simulink model "project"  (R2019a)
settings: Solver=FixedStepAuto  StartTime=0.0  StopTime=100  FixedStep=0.001  RelTol=1e-3
libraries: simulink x1
(part 1 of 2)
settings Model: Creator=shemmati  LastModifiedBy=shemmati
settings DataIOCC: ReturnWorkspaceOutputs=off
settings DebuggingCC: PregeneratedLibrarySubsystemCodeDiagnostic=none  ArithmeticOperatorsInVariantConditions=warning
settings SFSimCC: SimUseLocalCustomCode=off
settings RTWCC: RTWUseLocalCustomCode=off

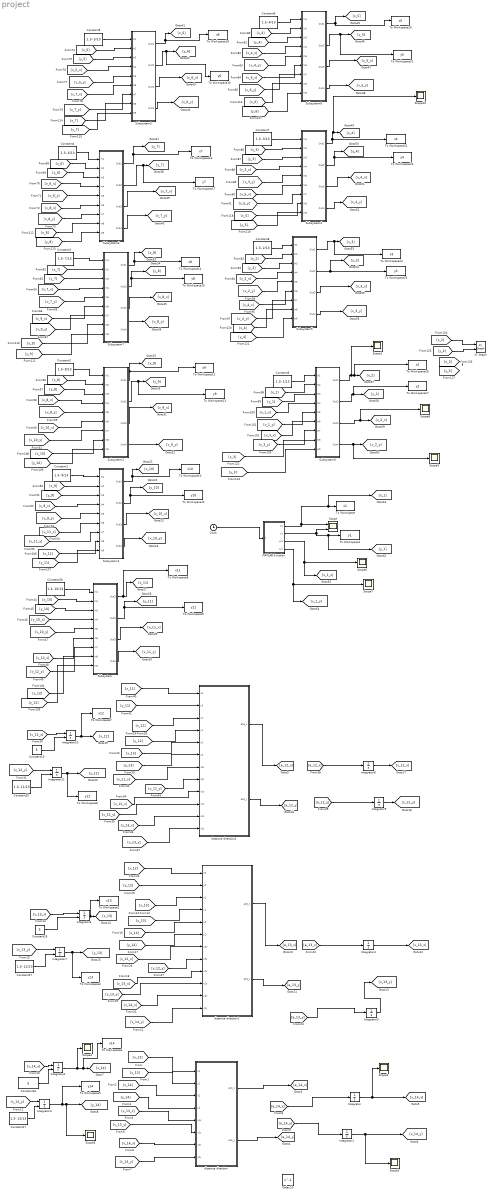
== system project ==
  Clock : Clock
  Constant1 : Constant  Value=1.3- 9/13
  Constant16 : Constant  Value=5
  Constant17 : Constant  Value=1.3- 13/13
  Constant18 : Constant  Value=5
  Constant19 : Constant  Value=5
  Constant2 : Constant  Value=1.3- 8/13
  Constant25 : Constant  Value=1.3- 11/13
  Constant27 : Constant  Value=1.3- 12/13
  Constant28 : Constant  Value=1.3- 10/13
  Constant3 : Constant  Value=1.3- 7/13
  Constant4 : Constant  Value=1.3- 6/13
  Constant5 : Constant  Value=1.3- 5/13
  Constant6 : Constant  Value=1.3- 4/13
  Constant7 : Constant  Value=1.3- 3/13
  Constant8 : Constant  Value=1.3- 2/13
  Constant9 : Constant  Value=1.3- 1/13
  Delay10 : Delay  DelayLength=1
  Integrator{,1,4..5,8..9} (6 alike) : Integrator
  Integrator{2..3,6..7,10..11} (6 alike) : Integrator  InitialConditionSource=external
  MATLAB Function : MATLAB Function  TreatAsAtomicUnit=on
  Scope : Scope  NumInputPorts=2
  Scope{1..10} (10 alike) : Scope
  Subsystem : Subsystem
  Subsystem1 : Subsystem
  Subsystem2 : Subsystem
  Subsystem3 : Subsystem
  Subsystem4 : Subsystem
  Subsystem5 : Subsystem
  Subsystem6 : Subsystem
  Subsystem7 : Subsystem
  Subsystem8 : Subsystem
  Subsystem9 : Subsystem
  To Workspace : ToWorkspace  VariableName=x1  SaveFormat=Timeseries  SampleTime=-1
  To Workspace1 : ToWorkspace  VariableName=y1  SaveFormat=Timeseries  SampleTime=-1
  To Workspace10 : ToWorkspace  VariableName=x10  SaveFormat=Timeseries  SampleTime=-1
  To Workspace11 : ToWorkspace  VariableName=y10  SaveFormat=Timeseries  SampleTime=-1
  To Workspace12 : ToWorkspace  VariableName=x9  SaveFormat=Timeseries  SampleTime=-1
  To Workspace13 : ToWorkspace  VariableName=y9  SaveFormat=Timeseries  SampleTime=-1
  To Workspace14 : ToWorkspace  VariableName=x8  SaveFormat=Timeseries  SampleTime=-1
  To Workspace15 : ToWorkspace  VariableName=y8  SaveFormat=Timeseries  SampleTime=-1
  To Workspace16 : ToWorkspace  VariableName=x7  SaveFormat=Timeseries  SampleTime=-1
  To Workspace17 : ToWorkspace  VariableName=y7  SaveFormat=Timeseries  SampleTime=-1
  To Workspace18 : ToWorkspace  VariableName=x6  SaveFormat=Timeseries  SampleTime=-1
  To Workspace19 : ToWorkspace  VariableName=y6  SaveFormat=Timeseries  SampleTime=-1
  To Workspace2 : ToWorkspace  VariableName=x13  SaveFormat=Timeseries  SampleTime=-1
  To Workspace20 : ToWorkspace  VariableName=x5  SaveFormat=Timeseries  SampleTime=-1
  To Workspace21 : ToWorkspace  VariableName=y5  SaveFormat=Timeseries  SampleTime=-1
  To Workspace22 : ToWorkspace  VariableName=x4  SaveFormat=Timeseries  SampleTime=-1
  To Workspace23 : ToWorkspace  VariableName=y4  SaveFormat=Timeseries  SampleTime=-1
  To Workspace24 : ToWorkspace  VariableName=x3  SaveFormat=Timeseries  SampleTime=-1
  To Workspace25 : ToWorkspace  VariableName=y3  SaveFormat=Timeseries  SampleTime=-1
  To Workspace26 : ToWorkspace  VariableName=x2  SaveFormat=Timeseries  SampleTime=-1
  To Workspace27 : ToWorkspace  VariableName=y2  SaveFormat=Timeseries  SampleTime=-1
  To Workspace3 : ToWorkspace  VariableName=y13  SaveFormat=Timeseries  SampleTime=-1
  To Workspace4 : ToWorkspace  VariableName=x14  SaveFormat=Timeseries  SampleTime=-1
  To Workspace5 : ToWorkspace  VariableName=y14  SaveFormat=Timeseries  SampleTime=-1
  To Workspace6 : ToWorkspace  VariableName=y12  SaveFormat=Timeseries  SampleTime=-1
  To Workspace7 : ToWorkspace  VariableName=x12  SaveFormat=Timeseries  SampleTime=-1
  To Workspace8 : ToWorkspace  VariableName=x11  SaveFormat=Timeseries  SampleTime=-1
  To Workspace9 : ToWorkspace  VariableName=y11  SaveFormat=Timeseries  SampleTime=-1
  XY Graph : simulink/Sinks/XY Graph  xmin=-20  xmax=20  ymin=-20  ymax=20  st=-1
  distance direction : MATLAB Function  TreatAsAtomicUnit=on
  distance direction1 : MATLAB Function  TreatAsAtomicUnit=on
  distance direction2 : MATLAB Function  TreatAsAtomicUnit=on
  wires:
  [x_13] -> distance direction/1(x1)
  [y_13] -> distance direction/2(y1)
  [x_14] -> distance direction/3(x2)
  [y_14] -> distance direction/4(y2)
  [v_14_x] -> Integrator2/1
  Constant16/1 -> Integrator2/2
  [v_14_y] -> Integrator3/1
  Constant17/1 -> Integrator3/2
  [x_13] -> distance direction1/3(x1)
  distance direction1/2(a13_y) -> [a_13_y]
  [v_14_x] -> distance direction1/11(v2x)
  [v_14_y] -> distance direction1/12(v2y)
  Integrator5/1 -> [v_13_y]
  Integrator4/1 -> [v_13_x]
  [v_13_y] -> distance direction1/10(v1y)
  [v_13_x] -> distance direction1/9(v1x)
  distance direction1/1(a13_x) -> [a_13_x]
  [y_14] -> distance direction1/6(y2)
  [y_13] -> distance direction1/4(y1)
  [v_13_y] -> Integrator7/1
  [v_13_x] -> Integrator6/1
  Constant18/1 -> Integrator6/2
  Constant27/1 -> Integrator7/2
  Integrator6/1 -> To Workspace2/1, [x_13]
  [x_14] -> distance direction1/5(x2)
  [x_12] -> distance direction1/1(x0)
  [y_12] -> distance direction1/2(y0)
  [v_12_x] -> distance direction1/7(v0x)
  [v_12_y] -> distance direction1/8(v0y)
  Integrator10/1 -> To Workspace7/1, [x_12]
  [x_13] -> distance direction2/5(x2)
  Integrator11/1 -> To Workspace6/1, [y_12]
  [v_12_x] -> Integrator10/1
  [y_13] -> distance direction2/6(y2)
  Constant25/1 -> Integrator11/2
  [v_12_y] -> Integrator11/1
  [x_11] -> distance direction2/1(x0)
  [v_11_x] -> distance direction2/7(v0x)
  Constant19/1 -> Integrator10/2
  [v_12_x] -> distance direction2/9(v1x)
  distance direction2/1(a13_x) -> [a_12_x]
  Integrator8/1 -> [v_12_x]
  Integrator9/1 -> [v_12_y]
  [v_12_y] -> distance direction2/10(v1y)
  distance direction2/2(a13_y) -> [a_12_y]
  [v_13_y] -> distance direction2/12(v2y)
  [y_11] -> distance direction2/2(y0)
  [x_12] -> distance direction2/3(x1)
  [v_11_y] -> distance direction2/8(v0y)
  [y_12] -> distance direction2/4(y1)
  [v_13_x] -> distance direction2/11(v2x)
  Constant28/1 -> Subsystem/1(In1)
  Subsystem/1(Out1) -> To Workspace8/1, [x_11]
  Subsystem/2(Out2) -> To Workspace9/1, [y_11]
  Subsystem/3(Out3) -> [v_11_x]
  Subsystem/4(Out4) -> [v_11_y]
  [x_10] -> Subsystem/2(In2)
  [y_10] -> Subsystem/3(In3)
  [v_10_x] -> Subsystem/4(In4)
  [v_10_y] -> Subsystem/5(In5)
  [v_12_x] -> Subsystem/6(In6)
  [v_12_y] -> Subsystem/7(In7)
  Subsystem1/4(Out4) -> [v_10_y]
  Subsystem1/1(Out1) -> To Workspace10/1, [x_10]
  Subsystem1/3(Out3) -> [v_10_x]
  Subsystem1/2(Out2) -> To Workspace11/1, [y_10]
  [v_11_y] -> Subsystem1/7(In7)
  Subsystem2/4(Out4) -> [v_9_y]
  Subsystem2/2(Out2) -> To Workspace13/1, [y_9]
  Subsystem2/3(Out3) -> [v_9_x]
  Subsystem2/1(Out1) -> To Workspace12/1, [x_9]
  Subsystem7/2(Out2) -> To Workspace15/1, [y_8]
  Subsystem7/4(Out4) -> [v_8_y]
  Subsystem7/3(Out3) -> [v_8_x]
  Subsystem7/1(Out1) -> To Workspace14/1, [x_8]
  Subsystem6/1(Out1) -> To Workspace16/1, [x_7]
  Subsystem6/2(Out2) -> To Workspace17/1, [y_7]
  Subsystem6/4(Out4) -> [v_7_y]
  Subsystem6/3(Out3) -> [v_7_x]
  Subsystem3/3(Out3) -> [v_6_x]
  Subsystem3/2(Out2) -> To Workspace19/1, [y_6]
  Subsystem3/1(Out1) -> To Workspace18/1, [x_6]
  Subsystem3/4(Out4) -> [v_6_y]
  Subsystem8/3(Out3) -> [v_5_x]
  Subsystem8/2(Out2) -> To Workspace21/1, [y_5]
  Subsystem8/1(Out1) -> [x_5], To Workspace20/1
  Subsystem8/4(Out4) -> [v_5_y]
  Subsystem5/1(Out1) -> To Workspace24/1, [x_3]
  Subsystem5/2(Out2) -> [y_3], To Workspace25/1
  Subsystem5/3(Out3) -> [v_3_x]
  Subsystem5/4(Out4) -> [v_3_y]
  MATLAB Function/2(y1) -> Scope/2, [y_1], To Workspace1/1
  Clock/1 -> MATLAB Function/1(t)
  MATLAB Function/1(x1) -> [x_1], To Workspace/1, Scope/1
  MATLAB Function/4(vy1) -> [v_1_y], Scope7/1
  MATLAB Function/3(vx1) -> Scope6/1, [v_1_x]
  [x_12] -> Subsystem/8(In8)
  [y_12] -> Subsystem/9(In9)
  Constant1/1 -> Subsystem1/1(In1)
  [x_9] -> Subsystem1/2(In2)
  [y_9] -> Subsystem1/3(In3)
  [v_9_x] -> Subsystem1/4(In4)
  [v_9_y] -> Subsystem1/5(In5)
  [v_11_x] -> Subsystem1/6(In6)
  [x_11] -> Subsystem1/8(In8)
  [y_11] -> Subsystem1/9(In9)
  Constant2/1 -> Subsystem2/1(In1)
  [x_8] -> Subsystem2/2(In2)
  [y_8] -> Subsystem2/3(In3)
  [v_8_x] -> Subsystem2/4(In4)
  [v_8_y] -> Subsystem2/5(In5)
  [v_10_x] -> Subsystem2/6(In6)
  [v_10_y] -> Subsystem2/7(In7)
  [x_10] -> Subsystem2/8(In8)
  [y_10] -> Subsystem2/9(In9)
  Constant3/1 -> Subsystem7/1(In1)
  [x_7] -> Subsystem7/2(In2)
  [y_7] -> Subsystem7/3(In3)
  [v_7_x] -> Subsystem7/4(In4)
  [v_7_y] -> Subsystem7/5(In5)
  [v_9_x] -> Subsystem7/6(In6)
  [v_9_y] -> Subsystem7/7(In7)
  [x_9] -> Subsystem7/8(In8)
  [y_9] -> Subsystem7/9(In9)
  [y_8] -> Subsystem6/9(In9)
  [x_8] -> Subsystem6/8(In8)
  [v_8_y] -> Subsystem6/7(In7)
  [v_8_x] -> Subsystem6/6(In6)
  [v_6_y] -> Subsystem6/5(In5)
  [v_6_x] -> Subsystem6/4(In4)
  [y_6] -> Subsystem6/3(In3)
  [x_6] -> Subsystem6/2(In2)
  Constant4/1 -> Subsystem6/1(In1)
  Constant5/1 -> Subsystem3/1(In1)
  [x_5] -> Subsystem3/2(In2)
  [y_5] -> Subsystem3/3(In3)
  [v_5_x] -> Subsystem3/4(In4)
  [v_5_y] -> Subsystem3/5(In5)
  [v_7_x] -> Subsystem3/6(In6)
  [v_7_y] -> Subsystem3/7(In7)
  [x_7] -> Subsystem3/8(In8)
  [y_7] -> Subsystem3/9(In9)
  Constant6/1 -> Subsystem8/1(In1)
  [x_4] -> Subsystem8/2(In2)
  [y_4] -> Subsystem8/3(In3)
  [v_4_x] -> Subsystem8/4(In4)
  [v_4_y] -> Subsystem8/5(In5)
  [v_6_x] -> Subsystem8/6(In6)
  [v_6_y] -> Subsystem8/7(In7)
  [x_6] -> Subsystem8/8(In8)
  [y_6] -> Subsystem8/9(In9)
  Constant7/1 -> Subsystem4/1(In1)
  [x_3] -> Subsystem4/2(In2)
  [y_3] -> Subsystem4/3(In3)
  [v_3_x] -> Subsystem4/4(In4)
  [v_3_y] -> Subsystem4/5(In5)
  [v_5_x] -> Subsystem4/6(In6)
  [v_5_y] -> Subsystem4/7(In7)
  [x_5] -> Subsystem4/8(In8)
  [y_5] -> Subsystem4/9(In9)
  Subsystem4/1(Out1) -> To Workspace22/1, Scope10/1, [x_4]
  Subsystem4/2(Out2) -> [y_4], To Workspace23/1
  Subsystem4/3(Out3) -> [v_4_x]
  Subsystem4/4(Out4) -> [v_4_y]
  Constant8/1 -> Subsystem5/1(In1)
  [x_2] -> Subsystem5/2(In2)
  [y_2] -> Subsystem5/3(In3)
  [v_2_x] -> Subsystem5/4(In4)
  [v_2_y] -> Subsystem5/5(In5)
  [v_4_x] -> Subsystem5/6(In6)
  [v_4_y] -> Subsystem5/7(In7)
  [x_4] -> Subsystem5/8(In8)
  [y_4] -> Subsystem5/9(In9)
  Constant9/1 -> Subsystem9/1(In1)
  [x_1] -> Subsystem9/2(In2)
  [y_1] -> Subsystem9/3(In3)
  [v_1_x] -> Subsystem9/4(In4)
  [v_1_y] -> Subsystem9/5(In5)
  [v_3_x] -> Subsystem9/6(In6)
  [v_3_y] -> Subsystem9/7(In7)
  Subsystem9/1(Out1) -> Scope1/1, To Workspace26/1, [x_2]
  Subsystem9/2(Out2) -> To Workspace27/1, [y_2]
  Subsystem9/3(Out3) -> Scope8/1, [v_2_x]
  Subsystem9/4(Out4) -> Scope9/1, [v_2_y]
  [x_3] -> Subsystem9/8(In8)
  [y_3] -> Subsystem9/9(In9)
  distance direction/1(a14_x) -> [a_14_x]
  distance direction/2(a14_y) -> [a_14_y]
  [v_14_y] -> distance direction/8(v2y)
  [v_14_x] -> distance direction/7(v2x)
  [v_13_y] -> distance direction/6(v1y)
  [v_13_x] -> distance direction/5(v1x)
  [a_13_x] -> Integrator4/1
  Integrator2/1 -> Scope4/1, To Workspace4/1, [x_14]
  Integrator3/1 -> To Workspace5/1, Scope5/1, [y_14]
  Integrator/1 -> Scope2/1, [v_14_x]
  Integrator1/1 -> Scope3/1, [v_14_y]
  [a_13_y] -> Integrator5/1
  [a_12_y] -> Integrator9/1
  [a_12_x] -> Integrator8/1
  [a_14_x] -> Integrator/1
  [a_14_y] -> Integrator1/1
  Integrator7/1 -> To Workspace3/1, [y_13]
  [x_2] -> XY Graph/1
  [y_2] -> XY Graph/2
  [x_3] -> ?

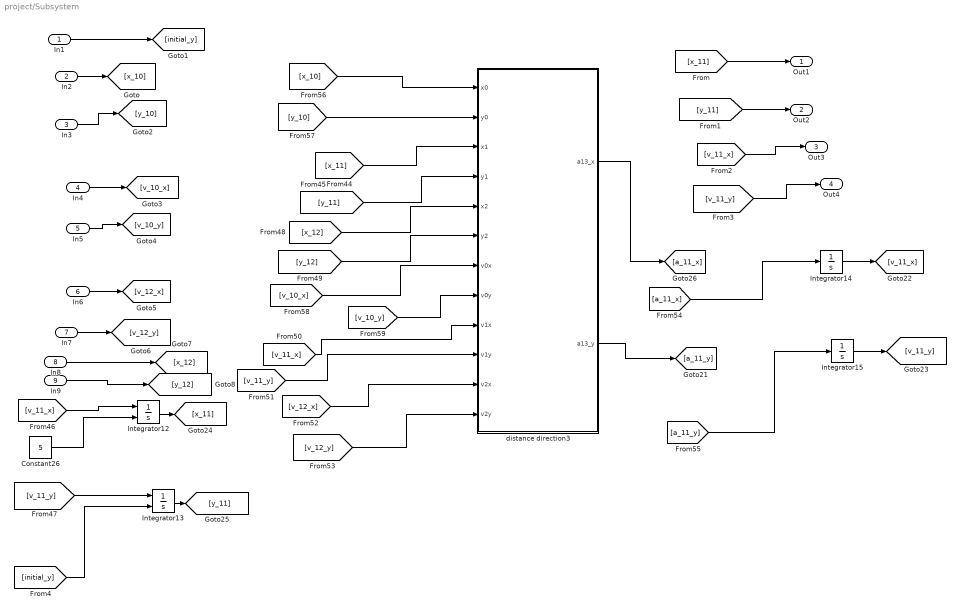
== system project/Subsystem ==
  In1 : Inport
  In2 : Inport  Port=2
  In3 : Inport  Port=3
  In4 : Inport  Port=4
  In5 : Inport  Port=5
  In6 : Inport  Port=6
  In7 : Inport  Port=7
  In8 : Inport  Port=8
  In9 : Inport  Port=9
  Constant26 : Constant  Value=5
  Integrator12 : Integrator  InitialConditionSource=external
  Integrator13 : Integrator  InitialConditionSource=external
  Integrator14 : Integrator
  Integrator15 : Integrator
  distance direction3 : MATLAB Function  TreatAsAtomicUnit=on
  Out1 : Outport
  Out2 : Outport  Port=2
  Out3 : Outport  Port=3
  Out4 : Outport  Port=4
  wires:
  distance direction3/1(a13_x) -> [a_11_x]
  Integrator15/1 -> [v_11_y]
  [v_12_y] -> distance direction3/12(v2y)
  [v_11_x] -> distance direction3/9(v1x)
  [v_10_x] -> distance direction3/7(v0x)
  distance direction3/2(a13_y) -> [a_11_y]
  [x_12] -> distance direction3/5(x2)
  [y_10] -> distance direction3/2(y0)
  [v_11_y] -> distance direction3/10(v1y)
  Constant26/1 -> Integrator12/2
  [v_12_x] -> distance direction3/11(v2x)
  [x_11] -> distance direction3/3(x1)
  [y_11] -> distance direction3/4(y1)
  Integrator12/1 -> [x_11]
  Integrator13/1 -> [y_11]
  [x_10] -> distance direction3/1(x0)
  [v_11_y] -> Integrator13/1
  Integrator14/1 -> [v_11_x]
  [initial_y] -> Integrator13/2
  [y_12] -> distance direction3/6(y2)
  [v_10_y] -> distance direction3/8(v0y)
  [v_11_x] -> Integrator12/1
  [x_11] -> Out1/1
  [y_11] -> Out2/1
  [v_11_x] -> Out3/1
  [v_11_y] -> Out4/1
  In1/1 -> [initial_y]
  In2/1 -> [x_10]
  In3/1 -> [y_10]
  In4/1 -> [v_10_x]
  In5/1 -> [v_10_y]
  In6/1 -> [v_12_x]
  In7/1 -> [v_12_y]
  In8/1 -> [x_12]
  In9/1 -> [y_12]
  [a_11_x] -> Integrator14/1
  [a_11_y] -> Integrator15/1

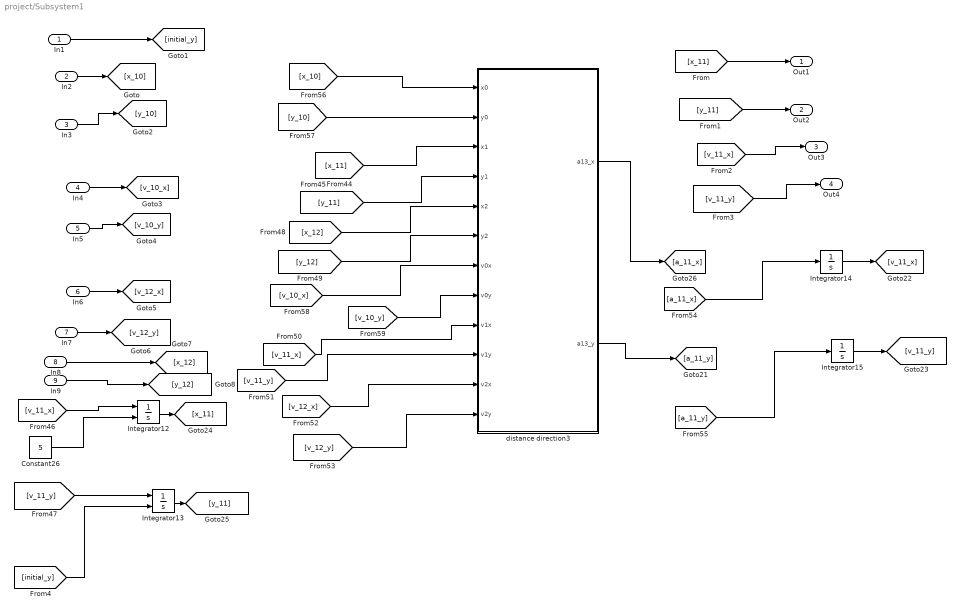
== system project/Subsystem1 ==
  In1 : Inport
  In2 : Inport  Port=2
  In3 : Inport  Port=3
  In4 : Inport  Port=4
  In5 : Inport  Port=5
  In6 : Inport  Port=6
  In7 : Inport  Port=7
  In8 : Inport  Port=8
  In9 : Inport  Port=9
  Constant26 : Constant  Value=5
  Integrator12 : Integrator  InitialConditionSource=external
  Integrator13 : Integrator  InitialConditionSource=external
  Integrator14 : Integrator
  Integrator15 : Integrator
  distance direction3 : MATLAB Function  TreatAsAtomicUnit=on
  Out1 : Outport
  Out2 : Outport  Port=2
  Out3 : Outport  Port=3
  Out4 : Outport  Port=4
  wires:
  distance direction3/1(a13_x) -> [a_11_x]
  Integrator15/1 -> [v_11_y]
  [v_12_y] -> distance direction3/12(v2y)
  [v_11_x] -> distance direction3/9(v1x)
  [v_10_x] -> distance direction3/7(v0x)
  distance direction3/2(a13_y) -> [a_11_y]
  [x_12] -> distance direction3/5(x2)
  [y_10] -> distance direction3/2(y0)
  [v_11_y] -> distance direction3/10(v1y)
  Constant26/1 -> Integrator12/2
  [v_12_x] -> distance direction3/11(v2x)
  [x_11] -> distance direction3/3(x1)
  [y_11] -> distance direction3/4(y1)
  Integrator12/1 -> [x_11]
  Integrator13/1 -> [y_11]
  [x_10] -> distance direction3/1(x0)
  [v_11_y] -> Integrator13/1
  Integrator14/1 -> [v_11_x]
  [initial_y] -> Integrator13/2
  [y_12] -> distance direction3/6(y2)
  [v_10_y] -> distance direction3/8(v0y)
  [v_11_x] -> Integrator12/1
  [x_11] -> Out1/1
  [y_11] -> Out2/1
  [v_11_x] -> Out3/1
  [v_11_y] -> Out4/1
  In1/1 -> [initial_y]
  In2/1 -> [x_10]
  In3/1 -> [y_10]
  In4/1 -> [v_10_x]
  In5/1 -> [v_10_y]
  In6/1 -> [v_12_x]
  In7/1 -> [v_12_y]
  In8/1 -> [x_12]
  In9/1 -> [y_12]
  [a_11_x] -> Integrator14/1
  [a_11_y] -> Integrator15/1

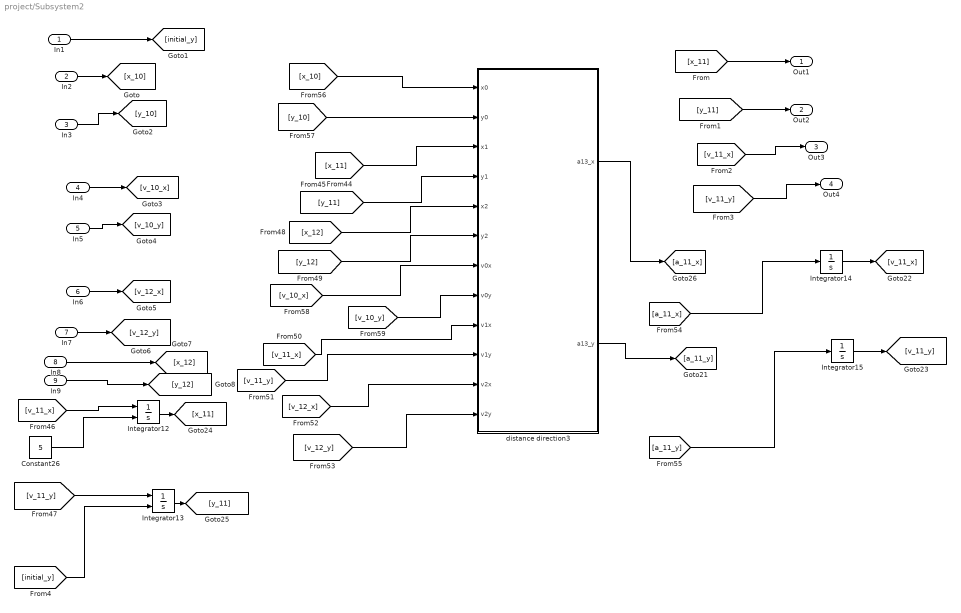
== system project/Subsystem2 ==
  In1 : Inport
  In2 : Inport  Port=2
  In3 : Inport  Port=3
  In4 : Inport  Port=4
  In5 : Inport  Port=5
  In6 : Inport  Port=6
  In7 : Inport  Port=7
  In8 : Inport  Port=8
  In9 : Inport  Port=9
  Constant26 : Constant  Value=5
  Integrator12 : Integrator  InitialConditionSource=external
  Integrator13 : Integrator  InitialConditionSource=external
  Integrator14 : Integrator
  Integrator15 : Integrator
  distance direction3 : MATLAB Function  TreatAsAtomicUnit=on
  Out1 : Outport
  Out2 : Outport  Port=2
  Out3 : Outport  Port=3
  Out4 : Outport  Port=4
  wires:
  distance direction3/1(a13_x) -> [a_11_x]
  Integrator15/1 -> [v_11_y]
  [v_12_y] -> distance direction3/12(v2y)
  [v_11_x] -> distance direction3/9(v1x)
  [v_10_x] -> distance direction3/7(v0x)
  distance direction3/2(a13_y) -> [a_11_y]
  [x_12] -> distance direction3/5(x2)
  [y_10] -> distance direction3/2(y0)
  [v_11_y] -> distance direction3/10(v1y)
  Constant26/1 -> Integrator12/2
  [v_12_x] -> distance direction3/11(v2x)
  [x_11] -> distance direction3/3(x1)
  [y_11] -> distance direction3/4(y1)
  Integrator12/1 -> [x_11]
  Integrator13/1 -> [y_11]
  [x_10] -> distance direction3/1(x0)
  [v_11_y] -> Integrator13/1
  Integrator14/1 -> [v_11_x]
  [initial_y] -> Integrator13/2
  [y_12] -> distance direction3/6(y2)
  [v_10_y] -> distance direction3/8(v0y)
  [v_11_x] -> Integrator12/1
  [x_11] -> Out1/1
  [y_11] -> Out2/1
  [v_11_x] -> Out3/1
  [v_11_y] -> Out4/1
  In1/1 -> [initial_y]
  In2/1 -> [x_10]
  In3/1 -> [y_10]
  In4/1 -> [v_10_x]
  In5/1 -> [v_10_y]
  In6/1 -> [v_12_x]
  In7/1 -> [v_12_y]
  In8/1 -> [x_12]
  In9/1 -> [y_12]
  [a_11_x] -> Integrator14/1
  [a_11_y] -> Integrator15/1

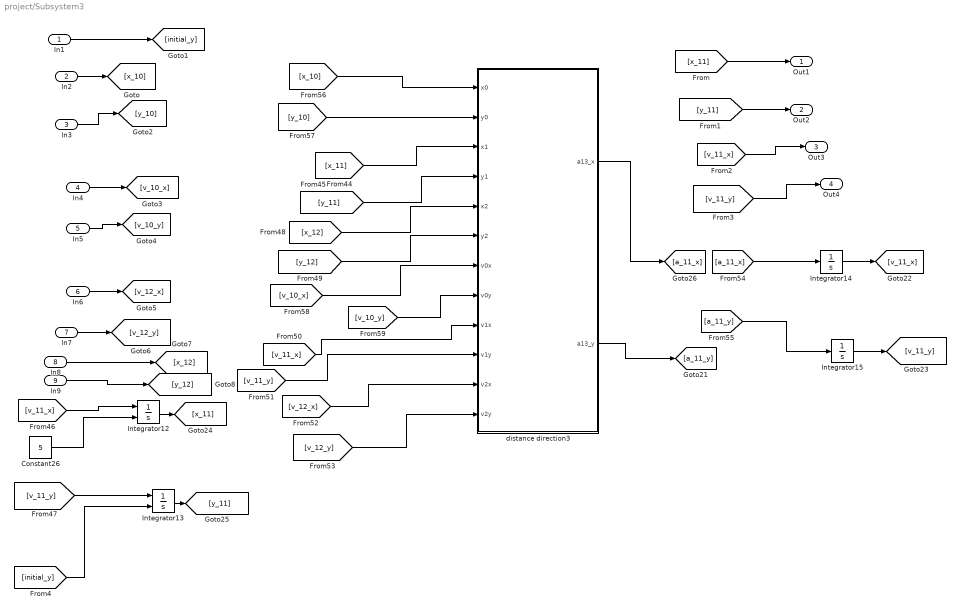
== system project/Subsystem3 ==
  In1 : Inport
  In2 : Inport  Port=2
  In3 : Inport  Port=3
  In4 : Inport  Port=4
  In5 : Inport  Port=5
  In6 : Inport  Port=6
  In7 : Inport  Port=7
  In8 : Inport  Port=8
  In9 : Inport  Port=9
  Constant26 : Constant  Value=5
  Integrator12 : Integrator  InitialConditionSource=external
  Integrator13 : Integrator  InitialConditionSource=external
  Integrator14 : Integrator
  Integrator15 : Integrator
  distance direction3 : MATLAB Function  TreatAsAtomicUnit=on
  Out1 : Outport
  Out2 : Outport  Port=2
  Out3 : Outport  Port=3
  Out4 : Outport  Port=4
  wires:
  distance direction3/1(a13_x) -> [a_11_x]
  Integrator15/1 -> [v_11_y]
  [v_12_y] -> distance direction3/12(v2y)
  [v_11_x] -> distance direction3/9(v1x)
  [v_10_x] -> distance direction3/7(v0x)
  distance direction3/2(a13_y) -> [a_11_y]
  [x_12] -> distance direction3/5(x2)
  [y_10] -> distance direction3/2(y0)
  [v_11_y] -> distance direction3/10(v1y)
  Constant26/1 -> Integrator12/2
  [v_12_x] -> distance direction3/11(v2x)
  [x_11] -> distance direction3/3(x1)
  [y_11] -> distance direction3/4(y1)
  Integrator12/1 -> [x_11]
  Integrator13/1 -> [y_11]
  [x_10] -> distance direction3/1(x0)
  [v_11_y] -> Integrator13/1
  Integrator14/1 -> [v_11_x]
  [initial_y] -> Integrator13/2
  [y_12] -> distance direction3/6(y2)
  [v_10_y] -> distance direction3/8(v0y)
  [v_11_x] -> Integrator12/1
  [x_11] -> Out1/1
  [y_11] -> Out2/1
  [v_11_x] -> Out3/1
  [v_11_y] -> Out4/1
  In1/1 -> [initial_y]
  In2/1 -> [x_10]
  In3/1 -> [y_10]
  In4/1 -> [v_10_x]
  In5/1 -> [v_10_y]
  In6/1 -> [v_12_x]
  In7/1 -> [v_12_y]
  In8/1 -> [x_12]
  In9/1 -> [y_12]
  [a_11_x] -> Integrator14/1
  [a_11_y] -> Integrator15/1

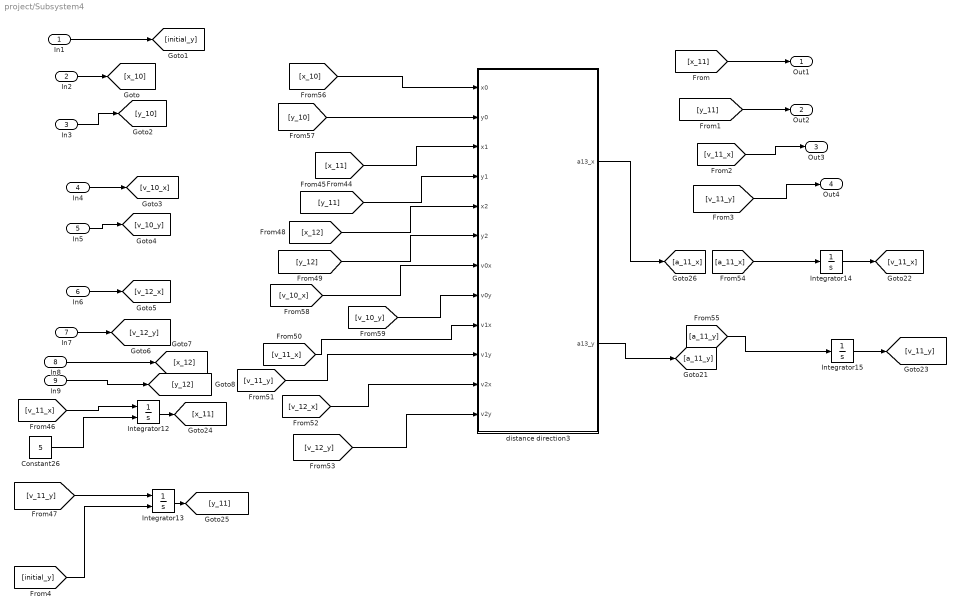
== system project/Subsystem4 ==
  In1 : Inport
  In2 : Inport  Port=2
  In3 : Inport  Port=3
  In4 : Inport  Port=4
  In5 : Inport  Port=5
  In6 : Inport  Port=6
  In7 : Inport  Port=7
  In8 : Inport  Port=8
  In9 : Inport  Port=9
  Constant26 : Constant  Value=5
  Integrator12 : Integrator  InitialConditionSource=external
  Integrator13 : Integrator  InitialConditionSource=external
  Integrator14 : Integrator
  Integrator15 : Integrator
  distance direction3 : MATLAB Function  TreatAsAtomicUnit=on
  Out1 : Outport
  Out2 : Outport  Port=2
  Out3 : Outport  Port=3
  Out4 : Outport  Port=4
  wires:
  distance direction3/1(a13_x) -> [a_11_x]
  Integrator15/1 -> [v_11_y]
  [v_12_y] -> distance direction3/12(v2y)
  [v_11_x] -> distance direction3/9(v1x)
  [v_10_x] -> distance direction3/7(v0x)
  distance direction3/2(a13_y) -> [a_11_y]
  [x_12] -> distance direction3/5(x2)
  [y_10] -> distance direction3/2(y0)
  [v_11_y] -> distance direction3/10(v1y)
  Constant26/1 -> Integrator12/2
  [v_12_x] -> distance direction3/11(v2x)
  [x_11] -> distance direction3/3(x1)
  [y_11] -> distance direction3/4(y1)
  Integrator12/1 -> [x_11]
  Integrator13/1 -> [y_11]
  [x_10] -> distance direction3/1(x0)
  [v_11_y] -> Integrator13/1
  Integrator14/1 -> [v_11_x]
  [initial_y] -> Integrator13/2
  [y_12] -> distance direction3/6(y2)
  [v_10_y] -> distance direction3/8(v0y)
  [v_11_x] -> Integrator12/1
  [x_11] -> Out1/1
  [y_11] -> Out2/1
  [v_11_x] -> Out3/1
  [v_11_y] -> Out4/1
  In1/1 -> [initial_y]
  In2/1 -> [x_10]
  In3/1 -> [y_10]
  In4/1 -> [v_10_x]
  In5/1 -> [v_10_y]
  In6/1 -> [v_12_x]
  In7/1 -> [v_12_y]
  In8/1 -> [x_12]
  In9/1 -> [y_12]
  [a_11_x] -> Integrator14/1
  [a_11_y] -> Integrator15/1

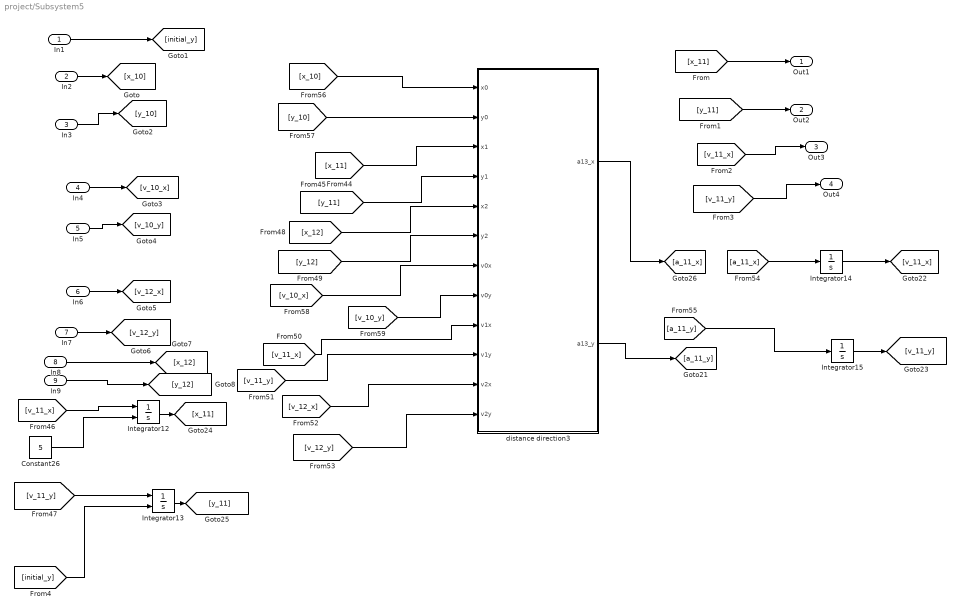
== system project/Subsystem5 ==
  In1 : Inport
  In2 : Inport  Port=2
  In3 : Inport  Port=3
  In4 : Inport  Port=4
  In5 : Inport  Port=5
  In6 : Inport  Port=6
  In7 : Inport  Port=7
  In8 : Inport  Port=8
  In9 : Inport  Port=9
  Constant26 : Constant  Value=5
  Integrator12 : Integrator  InitialConditionSource=external
  Integrator13 : Integrator  InitialConditionSource=external
  Integrator14 : Integrator
  Integrator15 : Integrator
  distance direction3 : MATLAB Function  TreatAsAtomicUnit=on
  Out1 : Outport
  Out2 : Outport  Port=2
  Out3 : Outport  Port=3
  Out4 : Outport  Port=4
  wires:
  distance direction3/1(a13_x) -> [a_11_x]
  Integrator15/1 -> [v_11_y]
  [v_12_y] -> distance direction3/12(v2y)
  [v_11_x] -> distance direction3/9(v1x)
  [v_10_x] -> distance direction3/7(v0x)
  distance direction3/2(a13_y) -> [a_11_y]
  [x_12] -> distance direction3/5(x2)
  [y_10] -> distance direction3/2(y0)
  [v_11_y] -> distance direction3/10(v1y)
  Constant26/1 -> Integrator12/2
  [v_12_x] -> distance direction3/11(v2x)
  [x_11] -> distance direction3/3(x1)
  [y_11] -> distance direction3/4(y1)
  Integrator12/1 -> [x_11]
  Integrator13/1 -> [y_11]
  [x_10] -> distance direction3/1(x0)
  [v_11_y] -> Integrator13/1
  Integrator14/1 -> [v_11_x]
  [initial_y] -> Integrator13/2
  [y_12] -> distance direction3/6(y2)
  [v_10_y] -> distance direction3/8(v0y)
  [v_11_x] -> Integrator12/1
  [x_11] -> Out1/1
  [y_11] -> Out2/1
  [v_11_x] -> Out3/1
  [v_11_y] -> Out4/1
  In1/1 -> [initial_y]
  In2/1 -> [x_10]
  In3/1 -> [y_10]
  In4/1 -> [v_10_x]
  In5/1 -> [v_10_y]
  In6/1 -> [v_12_x]
  In7/1 -> [v_12_y]
  In8/1 -> [x_12]
  In9/1 -> [y_12]
  [a_11_x] -> Integrator14/1
  [a_11_y] -> Integrator15/1

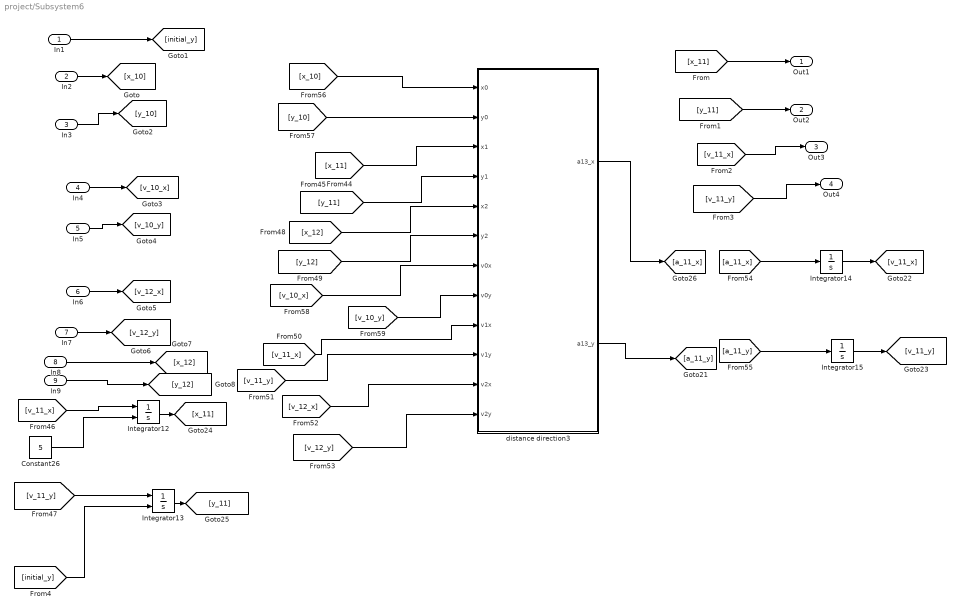
== system project/Subsystem6 ==
  In1 : Inport
  In2 : Inport  Port=2
  In3 : Inport  Port=3
  In4 : Inport  Port=4
  In5 : Inport  Port=5
  In6 : Inport  Port=6
  In7 : Inport  Port=7
  In8 : Inport  Port=8
  In9 : Inport  Port=9
  Constant26 : Constant  Value=5
  Integrator12 : Integrator  InitialConditionSource=external
  Integrator13 : Integrator  InitialConditionSource=external
  Integrator14 : Integrator
  Integrator15 : Integrator
  distance direction3 : MATLAB Function  TreatAsAtomicUnit=on
  Out1 : Outport
  Out2 : Outport  Port=2
  Out3 : Outport  Port=3
  Out4 : Outport  Port=4
  wires:
  distance direction3/1(a13_x) -> [a_11_x]
  Integrator15/1 -> [v_11_y]
  [v_12_y] -> distance direction3/12(v2y)
  [v_11_x] -> distance direction3/9(v1x)
  [v_10_x] -> distance direction3/7(v0x)
  distance direction3/2(a13_y) -> [a_11_y]
  [x_12] -> distance direction3/5(x2)
  [y_10] -> distance direction3/2(y0)
  [v_11_y] -> distance direction3/10(v1y)
  Constant26/1 -> Integrator12/2
  [v_12_x] -> distance direction3/11(v2x)
  [x_11] -> distance direction3/3(x1)
  [y_11] -> distance direction3/4(y1)
  Integrator12/1 -> [x_11]
  Integrator13/1 -> [y_11]
  [x_10] -> distance direction3/1(x0)
  [v_11_y] -> Integrator13/1
  Integrator14/1 -> [v_11_x]
  [initial_y] -> Integrator13/2
  [y_12] -> distance direction3/6(y2)
  [v_10_y] -> distance direction3/8(v0y)
  [v_11_x] -> Integrator12/1
  [x_11] -> Out1/1
  [y_11] -> Out2/1
  [v_11_x] -> Out3/1
  [v_11_y] -> Out4/1
  In1/1 -> [initial_y]
  In2/1 -> [x_10]
  In3/1 -> [y_10]
  In4/1 -> [v_10_x]
  In5/1 -> [v_10_y]
  In6/1 -> [v_12_x]
  In7/1 -> [v_12_y]
  In8/1 -> [x_12]
  In9/1 -> [y_12]
  [a_11_x] -> Integrator14/1
  [a_11_y] -> Integrator15/1

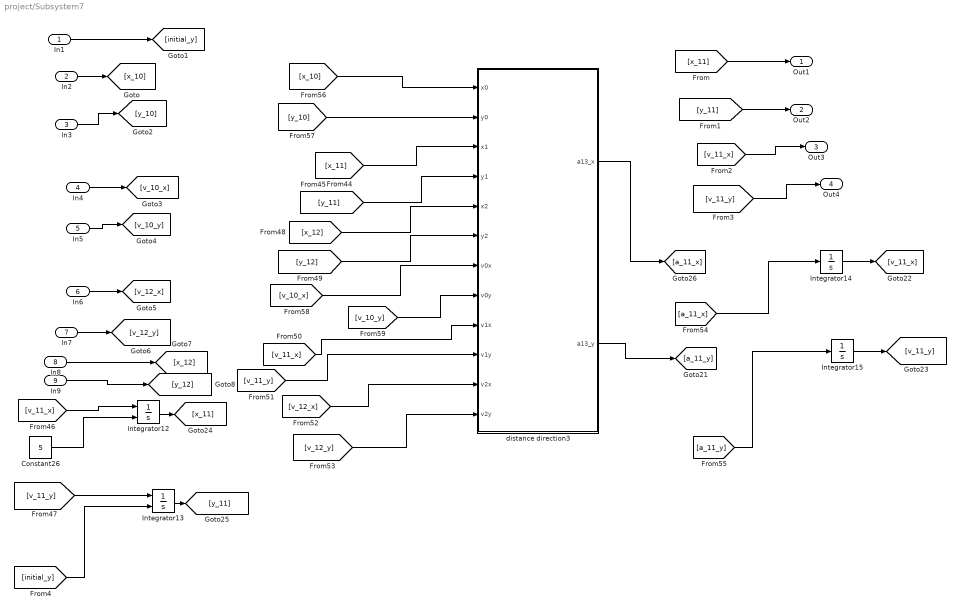
== system project/Subsystem7 ==
  In1 : Inport
  In2 : Inport  Port=2
  In3 : Inport  Port=3
  In4 : Inport  Port=4
  In5 : Inport  Port=5
  In6 : Inport  Port=6
  In7 : Inport  Port=7
  In8 : Inport  Port=8
  In9 : Inport  Port=9
  Constant26 : Constant  Value=5
  Integrator12 : Integrator  InitialConditionSource=external
  Integrator13 : Integrator  InitialConditionSource=external
  Integrator14 : Integrator
  Integrator15 : Integrator
  distance direction3 : MATLAB Function  TreatAsAtomicUnit=on
  Out1 : Outport
  Out2 : Outport  Port=2
  Out3 : Outport  Port=3
  Out4 : Outport  Port=4
  wires:
  distance direction3/1(a13_x) -> [a_11_x]
  Integrator15/1 -> [v_11_y]
  [v_12_y] -> distance direction3/12(v2y)
  [v_11_x] -> distance direction3/9(v1x)
  [v_10_x] -> distance direction3/7(v0x)
  distance direction3/2(a13_y) -> [a_11_y]
  [x_12] -> distance direction3/5(x2)
  [y_10] -> distance direction3/2(y0)
  [v_11_y] -> distance direction3/10(v1y)
  Constant26/1 -> Integrator12/2
  [v_12_x] -> distance direction3/11(v2x)
  [x_11] -> distance direction3/3(x1)
  [y_11] -> distance direction3/4(y1)
  Integrator12/1 -> [x_11]
  Integrator13/1 -> [y_11]
  [x_10] -> distance direction3/1(x0)
  [v_11_y] -> Integrator13/1
  Integrator14/1 -> [v_11_x]
  [initial_y] -> Integrator13/2
  [y_12] -> distance direction3/6(y2)
  [v_10_y] -> distance direction3/8(v0y)
  [v_11_x] -> Integrator12/1
  [x_11] -> Out1/1
  [y_11] -> Out2/1
  [v_11_x] -> Out3/1
  [v_11_y] -> Out4/1
  In1/1 -> [initial_y]
  In2/1 -> [x_10]
  In3/1 -> [y_10]
  In4/1 -> [v_10_x]
  In5/1 -> [v_10_y]
  In6/1 -> [v_12_x]
  In7/1 -> [v_12_y]
  In8/1 -> [x_12]
  In9/1 -> [y_12]
  [a_11_y] -> Integrator15/1
  [a_11_x] -> Integrator14/1

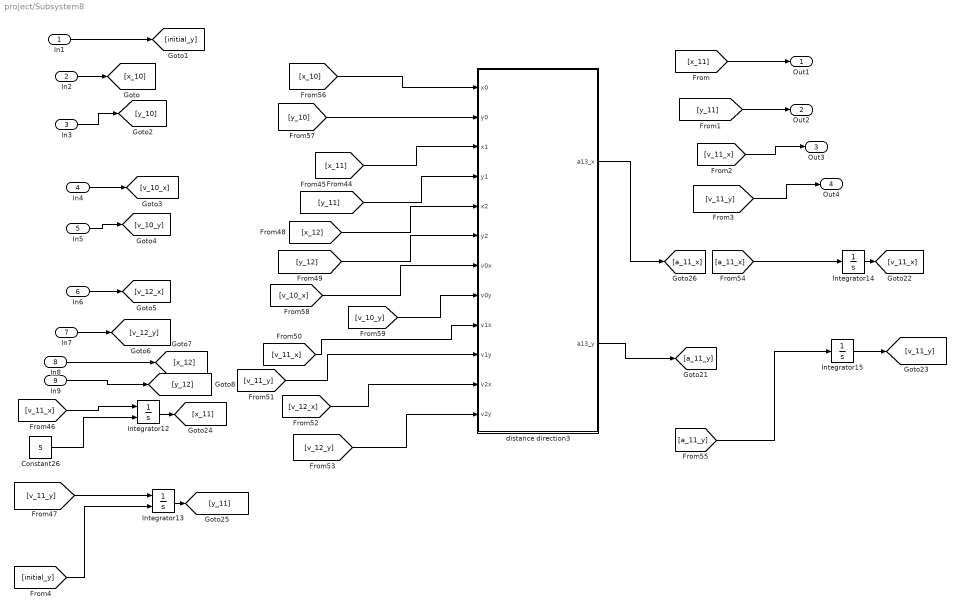
== system project/Subsystem8 ==
  In1 : Inport
  In2 : Inport  Port=2
  In3 : Inport  Port=3
  In4 : Inport  Port=4
  In5 : Inport  Port=5
  In6 : Inport  Port=6
  In7 : Inport  Port=7
  In8 : Inport  Port=8
  In9 : Inport  Port=9
  Constant26 : Constant  Value=5
  Integrator12 : Integrator  InitialConditionSource=external
  Integrator13 : Integrator  InitialConditionSource=external
  Integrator14 : Integrator
  Integrator15 : Integrator
  distance direction3 : MATLAB Function  TreatAsAtomicUnit=on
  Out1 : Outport
  Out2 : Outport  Port=2
  Out3 : Outport  Port=3
  Out4 : Outport  Port=4
  wires:
  distance direction3/1(a13_x) -> [a_11_x]
  Integrator15/1 -> [v_11_y]
  [v_12_y] -> distance direction3/12(v2y)
  [v_11_x] -> distance direction3/9(v1x)
  [v_10_x] -> distance direction3/7(v0x)
  distance direction3/2(a13_y) -> [a_11_y]
  [x_12] -> distance direction3/5(x2)
  [y_10] -> distance direction3/2(y0)
  [v_11_y] -> distance direction3/10(v1y)
  Constant26/1 -> Integrator12/2
  [v_12_x] -> distance direction3/11(v2x)
  [x_11] -> distance direction3/3(x1)
  [y_11] -> distance direction3/4(y1)
  Integrator12/1 -> [x_11]
  Integrator13/1 -> [y_11]
  [x_10] -> distance direction3/1(x0)
  [v_11_y] -> Integrator13/1
  Integrator14/1 -> [v_11_x]
  [initial_y] -> Integrator13/2
  [y_12] -> distance direction3/6(y2)
  [v_10_y] -> distance direction3/8(v0y)
  [v_11_x] -> Integrator12/1
  [x_11] -> Out1/1
  [y_11] -> Out2/1
  [v_11_x] -> Out3/1
  [v_11_y] -> Out4/1
  In1/1 -> [initial_y]
  In2/1 -> [x_10]
  In3/1 -> [y_10]
  In4/1 -> [v_10_x]
  In5/1 -> [v_10_y]
  In6/1 -> [v_12_x]
  In7/1 -> [v_12_y]
  In8/1 -> [x_12]
  In9/1 -> [y_12]
  [a_11_x] -> Integrator14/1
  [a_11_y] -> Integrator15/1

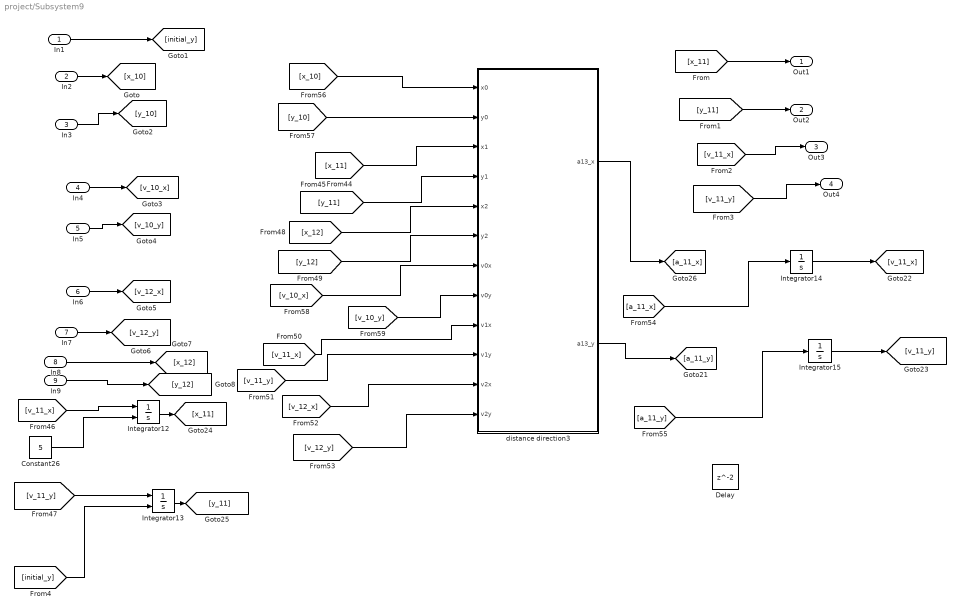
== system project/Subsystem9 ==
  In1 : Inport
  In2 : Inport  Port=2
  In3 : Inport  Port=3
  In4 : Inport  Port=4
  In5 : Inport  Port=5
  In6 : Inport  Port=6
  In7 : Inport  Port=7
  In8 : Inport  Port=8
  In9 : Inport  Port=9
  Constant26 : Constant  Value=5
  Delay : Delay
  Integrator12 : Integrator  InitialConditionSource=external
  Integrator13 : Integrator  InitialConditionSource=external
  Integrator14 : Integrator
  Integrator15 : Integrator
  distance direction3 : MATLAB Function  TreatAsAtomicUnit=on
  Out1 : Outport
  Out2 : Outport  Port=2
  Out3 : Outport  Port=3
  Out4 : Outport  Port=4
  wires:
  distance direction3/1(a13_x) -> [a_11_x]
  [v_12_y] -> distance direction3/12(v2y)
  [v_11_x] -> distance direction3/9(v1x)
  [v_10_x] -> distance direction3/7(v0x)
  distance direction3/2(a13_y) -> [a_11_y]
  [x_12] -> distance direction3/5(x2)
  [y_10] -> distance direction3/2(y0)
  [v_11_y] -> distance direction3/10(v1y)
  Constant26/1 -> Integrator12/2
  [v_12_x] -> distance direction3/11(v2x)
  [x_11] -> distance direction3/3(x1)
  [y_11] -> distance direction3/4(y1)
  Integrator12/1 -> [x_11]
  Integrator13/1 -> [y_11]
  [x_10] -> distance direction3/1(x0)
  [v_11_y] -> Integrator13/1
  [initial_y] -> Integrator13/2
  [y_12] -> distance direction3/6(y2)
  [v_10_y] -> distance direction3/8(v0y)
  [v_11_x] -> Integrator12/1
  [x_11] -> Out1/1
  [y_11] -> Out2/1
  [v_11_x] -> Out3/1
  [v_11_y] -> Out4/1
  In1/1 -> [initial_y]
  In2/1 -> [x_10]
  In3/1 -> [y_10]
  In4/1 -> [v_10_x]
  In5/1 -> [v_10_y]
  In6/1 -> [v_12_x]
  In7/1 -> [v_12_y]
  In8/1 -> [x_12]
  In9/1 -> [y_12]
  Integrator14/1 -> [v_11_x]
  Integrator15/1 -> [v_11_y]
  [a_11_x] -> Integrator14/1
  [a_11_y] -> Integrator15/1

== matlab function project/distance direction ==
  data: x1 input; y1 input; x2 input; y2 input; v1x input; v1y input; a14_x output size=1; a14_y output size=1; v2x input; v2y input
function [a14_x, a14_y] = fcn(x1, y1, x2, y2, v1x,v1y, v2x, v2y)




m=1/10;

k_s= 10;

k_d= 1;

L_r= 1/13;


distance= sqrt((x1-x2)^2 + (y1-y2)^2);


theta_after= atan2((y2-y1),(x2-x1));
% if x1~=x2
% theta_after= atan((y1-y2)/(x1-x2))
% else
% theta_after= 3.14/2;
% end


f_spring_x_13_14= -k_s* (distance - L_r)* cos(theta_after);

f_spring_y_13_14= -k_s* (distance - L_r)* sin(theta_after);



theta_damper_after= atan2((v2y-v1y),(v2x-v1x));
% if v1x~=v2x
% theta_damper_after= atan((v1y-v2y)/(v1x-v2x));
% else
% theta_damper_after= 3.14/2;
% end

damper_force= -k_d * (sqrt((v1y-v2y)^2 + (v1x-v2x)^2));



f_damper_x_13_14 = damper_force *cos(theta_damper_after);
f_damper_y_13_14 = damper_force *sin(theta_damper_after);




a14_x = (  f_spring_x_13_14  +   f_damper_x_13_14   )/m;

a14_y = (  f_spring_y_13_14  +   f_damper_y_13_14 + m* (-9.81)  )/m;

== matlab function project/MATLAB Function ==
  data: x1 output; t input; y1 output; vx1 output; vy1 output
function [x1,y1, vx1, vy1] = fcn(t)
m=1/10;

k_s= 10;

k_d= 1;

L_r= 1/13;

omega= 0.4 + 0.02 * t;
y1 = 1.3 + 5 * sin(omega*t);
x1= 5 * cos(omega*t);

vx1= -5 * sin(omega*t)* (0.4 + 0.04 * t);

vy1= 5 * cos(omega*t)* (0.4 + 0.04 * t);

== matlab function project/distance direction1 ==
  data: x0 input; y0 input; x1 input; y1 input; x2 input; y2 input; v0x input; v0y input; v1x input; v1y input; a13_x output; a13_y output; v2x input; v2y input
function [ a13_x, a13_y] = fcn(x0, y0, x1, y1, x2, y2, v0x, v0y, v1x,v1y, v2x, v2y)
m=1/10;

k_s= 10;

k_d= 1;

L_r= 1/13;

distance_13_14= sqrt((x1-x2)^2 + (y1-y2)^2);

distance_12_13= sqrt((x1-x0)^2 + (y1-y0)^2);




theta_after= atan2((y1-y2),(x1-x2));
% if x1~=x2
% theta_after= atan2((y1-y2),(x1-x2));
% else
% theta_after= 3.14/2;
% end

f_spring_x_13_14= -k_s* (distance_13_14 - L_r)* cos(theta_after);

f_spring_y_13_14= -k_s* (distance_13_14 - L_r)* sin(theta_after);



theta_before= atan2((y1-y0),(x1-x0));
% if x0~=x1
% theta_before= atan2((y0-y1),(x0-x1));
% else
% theta_before= 3.14/2;
% end

f_spring_x_12_13= -k_s* (distance_12_13 - L_r)* cos(theta_before);

f_spring_y_12_13= -k_s* (distance_12_13 - L_r)* sin(theta_before);






theta_damper_after= atan2((v1y-v2y),(v1x-v2x));
% if v1x~=v2x
% theta_damper_after= atan((v1y-v2y)/(v1x-v2x));
% else
% theta_damper_after= 3.14/2;
% end




damper_force= -k_d * (sqrt((v1y-v2y)^2 + (v1x-v2x)^2));

f_damper_x_13_14 = damper_force *cos(theta_damper_after);
f_damper_y_13_14 = damper_force *sin(theta_damper_after);




theta_damper_before= atan2((v1y-v0y),(v1x-v0x));
% if v0x~=v1x
% theta_damper_before= atan((v0y-v1y)/(v0x-v1x));
% else
% theta_damper_before= 3.14/2;
% end




damper_force_before= -k_d * (sqrt((v0y-v1y)^2 + (v0x-v1x)^2));

f_damper_x_12_13 = damper_force_before *cos(theta_damper_before);
f_damper_y_12_13 = damper_force_before *sin(theta_damper_before);







a13_x = (  f_spring_x_13_14  +   f_damper_x_13_14  + f_spring_x_12_13 + f_damper_x_12_13 )/m;

a13_y = (  f_spring_y_13_14  +   f_damper_y_13_14 + f_spring_y_12_13 + f_damper_y_12_13 + m* (-9.81)  )/m;

== matlab function project/distance direction2 ==
  data: x0 input; y0 input; x1 input; y1 input; x2 input; y2 input; v0x input; v0y input; v1x input; v1y input; a13_x output; a13_y output; v2x input; v2y input
function [ a13_x, a13_y] = fcn(x0, y0, x1, y1, x2, y2, v0x, v0y, v1x,v1y, v2x, v2y)
m=1/10;

k_s= 10;

k_d= 1;

L_r= 1/13;

distance_13_14= sqrt((x1-x2)^2 + (y1-y2)^2);

distance_12_13= sqrt((x1-x0)^2 + (y1-y0)^2);




theta_after= atan2((y1-y2),(x1-x2));
% if x1~=x2
% theta_after= atan2((y1-y2),(x1-x2));
% else
% theta_after= 3.14/2;
% end

f_spring_x_13_14= -k_s* (distance_13_14 - L_r)* cos(theta_after);

f_spring_y_13_14= -k_s* (distance_13_14 - L_r)* sin(theta_after);



theta_before= atan2((y1-y0),(x1-x0));
% if x0~=x1
% theta_before= atan2((y0-y1),(x0-x1));
% else
% theta_before= 3.14/2;
% end

f_spring_x_12_13= -k_s* (distance_12_13 - L_r)* cos(theta_before);

f_spring_y_12_13= -k_s* (distance_12_13 - L_r)* sin(theta_before);






theta_damper_after= atan2((v1y-v2y),(v1x-v2x));
% if v1x~=v2x
% theta_damper_after= atan((v1y-v2y)/(v1x-v2x));
% else
% theta_damper_after= 3.14/2;
% end




damper_force= -k_d * (sqrt((v1y-v2y)^2 + (v1x-v2x)^2));

f_damper_x_13_14 = damper_force *cos(theta_damper_after);
f_damper_y_13_14 = damper_force *sin(theta_damper_after);




theta_damper_before= atan2((v1y-v0y),(v1x-v0x));
% if v0x~=v1x
% theta_damper_before= atan((v0y-v1y)/(v0x-v1x));
% else
% theta_damper_before= 3.14/2;
% end




damper_force_before= -k_d * (sqrt((v0y-v1y)^2 + (v0x-v1x)^2));

f_damper_x_12_13 = damper_force_before *cos(theta_damper_before);
f_damper_y_12_13 = damper_force_before *sin(theta_damper_before);







a13_x = (  f_spring_x_13_14  +   f_damper_x_13_14  + f_spring_x_12_13 + f_damper_x_12_13 )/m;

a13_y = (  f_spring_y_13_14  +   f_damper_y_13_14 + f_spring_y_12_13 + f_damper_y_12_13 + m* (-9.81)  )/m;

== matlab function project/Subsystem1/distance direction3 ==
  data: x0 input; y0 input; x1 input; y1 input; x2 input; y2 input; v0x input; v0y input; v1x input; v1y input; a13_x output; a13_y output; v2x input; v2y input
function [ a13_x, a13_y] = fcn(x0, y0, x1, y1, x2, y2, v0x, v0y, v1x,v1y, v2x, v2y)
m=1/10;

k_s= 10;

k_d= 1;

L_r= 1/13;

distance_13_14= sqrt((x1-x2)^2 + (y1-y2)^2);

distance_12_13= sqrt((x1-x0)^2 + (y1-y0)^2);




theta_after= atan2((y1-y2),(x1-x2));
% if x1~=x2
% theta_after= atan2((y1-y2),(x1-x2));
% else
% theta_after= 3.14/2;
% end

f_spring_x_13_14= -k_s* (distance_13_14 - L_r)* cos(theta_after);

f_spring_y_13_14= -k_s* (distance_13_14 - L_r)* sin(theta_after);



theta_before= atan2((y1-y0),(x1-x0));
% if x0~=x1
% theta_before= atan2((y0-y1),(x0-x1));
% else
% theta_before= 3.14/2;
% end

f_spring_x_12_13= -k_s* (distance_12_13 - L_r)* cos(theta_before);

f_spring_y_12_13= -k_s* (distance_12_13 - L_r)* sin(theta_before);






theta_damper_after= atan2((v1y-v2y),(v1x-v2x));
% if v1x~=v2x
% theta_damper_after= atan((v1y-v2y)/(v1x-v2x));
% else
% theta_damper_after= 3.14/2;
% end




damper_force= -k_d * (sqrt((v1y-v2y)^2 + (v1x-v2x)^2));

f_damper_x_13_14 = damper_force *cos(theta_damper_after);
f_damper_y_13_14 = damper_force *sin(theta_damper_after);




theta_damper_before= atan2((v1y-v0y),(v1x-v0x));
% if v0x~=v1x
% theta_damper_before= atan((v0y-v1y)/(v0x-v1x));
% else
% theta_damper_before= 3.14/2;
% end




damper_force_before= -k_d * (sqrt((v0y-v1y)^2 + (v0x-v1x)^2));

f_damper_x_12_13 = damper_force_before *cos(theta_damper_before);
f_damper_y_12_13 = damper_force_before *sin(theta_damper_before);







a13_x = (  f_spring_x_13_14  +   f_damper_x_13_14  + f_spring_x_12_13 + f_damper_x_12_13 )/m;

a13_y = (  f_spring_y_13_14  +   f_damper_y_13_14 + f_spring_y_12_13 + f_damper_y_12_13 + m* (-9.81)  )/m;

== matlab function project/Subsystem/distance direction3 ==
  data: x0 input; y0 input; x1 input; y1 input; x2 input; y2 input; v0x input; v0y input; v1x input; v1y input; a13_x output; a13_y output; v2x input; v2y input
function [ a13_x, a13_y] = fcn(x0, y0, x1, y1, x2, y2, v0x, v0y, v1x,v1y, v2x, v2y)
m=1/10;

k_s= 10;

k_d= 1;

L_r= 1/13;

distance_13_14= sqrt((x1-x2)^2 + (y1-y2)^2);

distance_12_13= sqrt((x1-x0)^2 + (y1-y0)^2);




theta_after= atan2((y1-y2),(x1-x2));
% if x1~=x2
% theta_after= atan2((y1-y2),(x1-x2));
% else
% theta_after= 3.14/2;
% end

f_spring_x_13_14= -k_s* (distance_13_14 - L_r)* cos(theta_after);

f_spring_y_13_14= -k_s* (distance_13_14 - L_r)* sin(theta_after);



theta_before= atan2((y1-y0),(x1-x0));
% if x0~=x1
% theta_before= atan2((y0-y1),(x0-x1));
% else
% theta_before= 3.14/2;
% end

f_spring_x_12_13= -k_s* (distance_12_13 - L_r)* cos(theta_before);

f_spring_y_12_13= -k_s* (distance_12_13 - L_r)* sin(theta_before);






theta_damper_after= atan2((v1y-v2y),(v1x-v2x));
% if v1x~=v2x
% theta_damper_after= atan((v1y-v2y)/(v1x-v2x));
% else
% theta_damper_after= 3.14/2;
% end




damper_force= -k_d * (sqrt((v1y-v2y)^2 + (v1x-v2x)^2));

f_damper_x_13_14 = damper_force *cos(theta_damper_after);
f_damper_y_13_14 = damper_force *sin(theta_damper_after);




theta_damper_before= atan2((v1y-v0y),(v1x-v0x));
% if v0x~=v1x
% theta_damper_before= atan((v0y-v1y)/(v0x-v1x));
% else
% theta_damper_before= 3.14/2;
% end




damper_force_before= -k_d * (sqrt((v0y-v1y)^2 + (v0x-v1x)^2));

f_damper_x_12_13 = damper_force_before *cos(theta_damper_before);
f_damper_y_12_13 = damper_force_before *sin(theta_damper_before);







a13_x = (  f_spring_x_13_14  +   f_damper_x_13_14  + f_spring_x_12_13 + f_damper_x_12_13 )/m;

a13_y = (  f_spring_y_13_14  +   f_damper_y_13_14 + f_spring_y_12_13 + f_damper_y_12_13 + m* (-9.81)  )/m;

== matlab function project/Subsystem2/distance direction3 ==
  data: x0 input; y0 input; x1 input; y1 input; x2 input; y2 input; v0x input; v0y input; v1x input; v1y input; a13_x output; a13_y output; v2x input; v2y input
function [ a13_x, a13_y] = fcn(x0, y0, x1, y1, x2, y2, v0x, v0y, v1x,v1y, v2x, v2y)
m=1/10;

k_s= 10;

k_d= 1;

L_r= 1/13;

distance_13_14= sqrt((x1-x2)^2 + (y1-y2)^2);

distance_12_13= sqrt((x1-x0)^2 + (y1-y0)^2);




theta_after= atan2((y1-y2),(x1-x2));
% if x1~=x2
% theta_after= atan2((y1-y2),(x1-x2));
% else
% theta_after= 3.14/2;
% end

f_spring_x_13_14= -k_s* (distance_13_14 - L_r)* cos(theta_after);

f_spring_y_13_14= -k_s* (distance_13_14 - L_r)* sin(theta_after);



theta_before= atan2((y1-y0),(x1-x0));
% if x0~=x1
% theta_before= atan2((y0-y1),(x0-x1));
% else
% theta_before= 3.14/2;
% end

f_spring_x_12_13= -k_s* (distance_12_13 - L_r)* cos(theta_before);

f_spring_y_12_13= -k_s* (distance_12_13 - L_r)* sin(theta_before);






theta_damper_after= atan2((v1y-v2y),(v1x-v2x));
% if v1x~=v2x
% theta_damper_after= atan((v1y-v2y)/(v1x-v2x));
% else
% theta_damper_after= 3.14/2;
% end




damper_force= -k_d * (sqrt((v1y-v2y)^2 + (v1x-v2x)^2));

f_damper_x_13_14 = damper_force *cos(theta_damper_after);
f_damper_y_13_14 = damper_force *sin(theta_damper_after);




theta_damper_before= atan2((v1y-v0y),(v1x-v0x));
% if v0x~=v1x
% theta_damper_before= atan((v0y-v1y)/(v0x-v1x));
% else
% theta_damper_before= 3.14/2;
% end




damper_force_before= -k_d * (sqrt((v0y-v1y)^2 + (v0x-v1x)^2));

f_damper_x_12_13 = damper_force_before *cos(theta_damper_before);
f_damper_y_12_13 = damper_force_before *sin(theta_damper_before);







a13_x = (  f_spring_x_13_14  +   f_damper_x_13_14  + f_spring_x_12_13 + f_damper_x_12_13 )/m;

a13_y = (  f_spring_y_13_14  +   f_damper_y_13_14 + f_spring_y_12_13 + f_damper_y_12_13 + m* (-9.81)  )/m;

== matlab function project/Subsystem3/distance direction3 ==
  data: x0 input; y0 input; x1 input; y1 input; x2 input; y2 input; v0x input; v0y input; v1x input; v1y input; a13_x output; a13_y output; v2x input; v2y input
function [ a13_x, a13_y] = fcn(x0, y0, x1, y1, x2, y2, v0x, v0y, v1x,v1y, v2x, v2y)
m=1/10;

k_s= 10;

k_d= 1;

L_r= 1/13;

distance_13_14= sqrt((x1-x2)^2 + (y1-y2)^2);

distance_12_13= sqrt((x1-x0)^2 + (y1-y0)^2);




theta_after= atan2((y1-y2),(x1-x2));
% if x1~=x2
% theta_after= atan2((y1-y2),(x1-x2));
% else
% theta_after= 3.14/2;
% end

f_spring_x_13_14= -k_s* (distance_13_14 - L_r)* cos(theta_after);

f_spring_y_13_14= -k_s* (distance_13_14 - L_r)* sin(theta_after);



theta_before= atan2((y1-y0),(x1-x0));
% if x0~=x1
% theta_before= atan2((y0-y1),(x0-x1));
% else
% theta_before= 3.14/2;
% end

f_spring_x_12_13= -k_s* (distance_12_13 - L_r)* cos(theta_before);

f_spring_y_12_13= -k_s* (distance_12_13 - L_r)* sin(theta_before);






theta_damper_after= atan2((v1y-v2y),(v1x-v2x));
% if v1x~=v2x
% theta_damper_after= atan((v1y-v2y)/(v1x-v2x));
% else
% theta_damper_after= 3.14/2;
% end




damper_force= -k_d * (sqrt((v1y-v2y)^2 + (v1x-v2x)^2));

f_damper_x_13_14 = damper_force *cos(theta_damper_after);
f_damper_y_13_14 = damper_force *sin(theta_damper_after);




theta_damper_before= atan2((v1y-v0y),(v1x-v0x));
% if v0x~=v1x
% theta_damper_before= atan((v0y-v1y)/(v0x-v1x));
% else
% theta_damper_before= 3.14/2;
% end




damper_force_before= -k_d * (sqrt((v0y-v1y)^2 + (v0x-v1x)^2));

f_damper_x_12_13 = damper_force_before *cos(theta_damper_before);
f_damper_y_12_13 = damper_force_before *sin(theta_damper_before);







a13_x = (  f_spring_x_13_14  +   f_damper_x_13_14  + f_spring_x_12_13 + f_damper_x_12_13 )/m;

a13_y = (  f_spring_y_13_14  +   f_damper_y_13_14 + f_spring_y_12_13 + f_damper_y_12_13 + m* (-9.81)  )/m;

== matlab function project/Subsystem4/distance direction3 ==
  data: x0 input; y0 input; x1 input; y1 input; x2 input; y2 input; v0x input; v0y input; v1x input; v1y input; a13_x output; a13_y output; v2x input; v2y input
function [ a13_x, a13_y] = fcn(x0, y0, x1, y1, x2, y2, v0x, v0y, v1x,v1y, v2x, v2y)
m=1/10;

k_s= 10;

k_d= 1;

L_r= 1/13;

distance_13_14= sqrt((x1-x2)^2 + (y1-y2)^2);

distance_12_13= sqrt((x1-x0)^2 + (y1-y0)^2);




theta_after= atan2((y1-y2),(x1-x2));
% if x1~=x2
% theta_after= atan2((y1-y2),(x1-x2));
% else
% theta_after= 3.14/2;
% end

f_spring_x_13_14= -k_s* (distance_13_14 - L_r)* cos(theta_after);

f_spring_y_13_14= -k_s* (distance_13_14 - L_r)* sin(theta_after);



theta_before= atan2((y1-y0),(x1-x0));
% if x0~=x1
% theta_before= atan2((y0-y1),(x0-x1));
% else
% theta_before= 3.14/2;
% end

f_spring_x_12_13= -k_s* (distance_12_13 - L_r)* cos(theta_before);

f_spring_y_12_13= -k_s* (distance_12_13 - L_r)* sin(theta_before);






theta_damper_after= atan2((v1y-v2y),(v1x-v2x));
% if v1x~=v2x
% theta_damper_after= atan((v1y-v2y)/(v1x-v2x));
% else
% theta_damper_after= 3.14/2;
% end




damper_force= -k_d * (sqrt((v1y-v2y)^2 + (v1x-v2x)^2));

f_damper_x_13_14 = damper_force *cos(theta_damper_after);
f_damper_y_13_14 = damper_force *sin(theta_damper_after);




theta_damper_before= atan2((v1y-v0y),(v1x-v0x));
% if v0x~=v1x
% theta_damper_before= atan((v0y-v1y)/(v0x-v1x));
% else
% theta_damper_before= 3.14/2;
% end




damper_force_before= -k_d * (sqrt((v0y-v1y)^2 + (v0x-v1x)^2));

f_damper_x_12_13 = damper_force_before *cos(theta_damper_before);
f_damper_y_12_13 = damper_force_before *sin(theta_damper_before);







a13_x = (  f_spring_x_13_14  +   f_damper_x_13_14  + f_spring_x_12_13 + f_damper_x_12_13 )/m;

a13_y = (  f_spring_y_13_14  +   f_damper_y_13_14 + f_spring_y_12_13 + f_damper_y_12_13 + m* (-9.81)  )/m;

== matlab function project/Subsystem5/distance direction3 ==
  data: x0 input; y0 input; x1 input; y1 input; x2 input; y2 input; v0x input; v0y input; v1x input; v1y input; a13_x output; a13_y output; v2x input; v2y input
function [ a13_x, a13_y] = fcn(x0, y0, x1, y1, x2, y2, v0x, v0y, v1x,v1y, v2x, v2y)
m=1/10;

k_s= 10;

k_d= 1;

L_r= 1/13;

distance_13_14= sqrt((x1-x2)^2 + (y1-y2)^2);

distance_12_13= sqrt((x1-x0)^2 + (y1-y0)^2);




theta_after= atan2((y1-y2),(x1-x2));
% if x1~=x2
% theta_after= atan2((y1-y2),(x1-x2));
% else
% theta_after= 3.14/2;
% end

f_spring_x_13_14= -k_s* (distance_13_14 - L_r)* cos(theta_after);

f_spring_y_13_14= -k_s* (distance_13_14 - L_r)* sin(theta_after);



theta_before= atan2((y1-y0),(x1-x0));
% if x0~=x1
% theta_before= atan2((y0-y1),(x0-x1));
% else
% theta_before= 3.14/2;
% end

f_spring_x_12_13= -k_s* (distance_12_13 - L_r)* cos(theta_before);

f_spring_y_12_13= -k_s* (distance_12_13 - L_r)* sin(theta_before);






theta_damper_after= atan2((v1y-v2y),(v1x-v2x));
% if v1x~=v2x
% theta_damper_after= atan((v1y-v2y)/(v1x-v2x));
% else
% theta_damper_after= 3.14/2;
% end




damper_force= -k_d * (sqrt((v1y-v2y)^2 + (v1x-v2x)^2));

f_damper_x_13_14 = damper_force *cos(theta_damper_after);
f_damper_y_13_14 = damper_force *sin(theta_damper_after);




theta_damper_before= atan2((v1y-v0y),(v1x-v0x));
% if v0x~=v1x
% theta_damper_before= atan((v0y-v1y)/(v0x-v1x));
% else
% theta_damper_before= 3.14/2;
% end




damper_force_before= -k_d * (sqrt((v0y-v1y)^2 + (v0x-v1x)^2));

f_damper_x_12_13 = damper_force_before *cos(theta_damper_before);
f_damper_y_12_13 = damper_force_before *sin(theta_damper_before);







a13_x = (  f_spring_x_13_14  +   f_damper_x_13_14  + f_spring_x_12_13 + f_damper_x_12_13 )/m;

a13_y = (  f_spring_y_13_14  +   f_damper_y_13_14 + f_spring_y_12_13 + f_damper_y_12_13 + m* (-9.81)  )/m;

== matlab function project/Subsystem6/distance direction3 ==
  data: x0 input; y0 input; x1 input; y1 input; x2 input; y2 input; v0x input; v0y input; v1x input; v1y input; a13_x output; a13_y output; v2x input; v2y input
function [ a13_x, a13_y] = fcn(x0, y0, x1, y1, x2, y2, v0x, v0y, v1x,v1y, v2x, v2y)
m=1/10;

k_s= 10;

k_d= 1;

L_r= 1/13;

distance_13_14= sqrt((x1-x2)^2 + (y1-y2)^2);

distance_12_13= sqrt((x1-x0)^2 + (y1-y0)^2);




theta_after= atan2((y1-y2),(x1-x2));
% if x1~=x2
% theta_after= atan2((y1-y2),(x1-x2));
% else
% theta_after= 3.14/2;
% end

f_spring_x_13_14= -k_s* (distance_13_14 - L_r)* cos(theta_after);

f_spring_y_13_14= -k_s* (distance_13_14 - L_r)* sin(theta_after);



theta_before= atan2((y1-y0),(x1-x0));
% if x0~=x1
% theta_before= atan2((y0-y1),(x0-x1));
% else
% theta_before= 3.14/2;
% end

f_spring_x_12_13= -k_s* (distance_12_13 - L_r)* cos(theta_before);

f_spring_y_12_13= -k_s* (distance_12_13 - L_r)* sin(theta_before);






theta_damper_after= atan2((v1y-v2y),(v1x-v2x));
% if v1x~=v2x
% theta_damper_after= atan((v1y-v2y)/(v1x-v2x));
% else
% theta_damper_after= 3.14/2;
% end




damper_force= -k_d * (sqrt((v1y-v2y)^2 + (v1x-v2x)^2));

f_damper_x_13_14 = damper_force *cos(theta_damper_after);
f_damper_y_13_14 = damper_force *sin(theta_damper_after);




theta_damper_before= atan2((v1y-v0y),(v1x-v0x));
% if v0x~=v1x
% theta_damper_before= atan((v0y-v1y)/(v0x-v1x));
% else
% theta_damper_before= 3.14/2;
% end




damper_force_before= -k_d * (sqrt((v0y-v1y)^2 + (v0x-v1x)^2));

f_damper_x_12_13 = damper_force_before *cos(theta_damper_before);
f_damper_y_12_13 = damper_force_before *sin(theta_damper_before);







a13_x = (  f_spring_x_13_14  +   f_damper_x_13_14  + f_spring_x_12_13 + f_damper_x_12_13 )/m;

a13_y = (  f_spring_y_13_14  +   f_damper_y_13_14 + f_spring_y_12_13 + f_damper_y_12_13 + m* (-9.81)  )/m;

== matlab function project/Subsystem7/distance direction3 ==
  data: x0 input; y0 input; x1 input; y1 input; x2 input; y2 input; v0x input; v0y input; v1x input; v1y input; a13_x output; a13_y output; v2x input; v2y input
function [ a13_x, a13_y] = fcn(x0, y0, x1, y1, x2, y2, v0x, v0y, v1x,v1y, v2x, v2y)
m=1/10;

k_s= 10;

k_d= 1;

L_r= 1/13;

distance_13_14= sqrt((x1-x2)^2 + (y1-y2)^2);

distance_12_13= sqrt((x1-x0)^2 + (y1-y0)^2);




theta_after= atan2((y1-y2),(x1-x2));
% if x1~=x2
% theta_after= atan2((y1-y2),(x1-x2));
% else
% theta_after= 3.14/2;
% end

f_spring_x_13_14= -k_s* (distance_13_14 - L_r)* cos(theta_after);

f_spring_y_13_14= -k_s* (distance_13_14 - L_r)* sin(theta_after);



theta_before= atan2((y1-y0),(x1-x0));
% if x0~=x1
% theta_before= atan2((y0-y1),(x0-x1));
% else
% theta_before= 3.14/2;
% end

f_spring_x_12_13= -k_s* (distance_12_13 - L_r)* cos(theta_before);

f_spring_y_12_13= -k_s* (distance_12_13 - L_r)* sin(theta_before);






theta_damper_after= atan2((v1y-v2y),(v1x-v2x));
% if v1x~=v2x
% theta_damper_after= atan((v1y-v2y)/(v1x-v2x));
% else
% theta_damper_after= 3.14/2;
% end




damper_force= -k_d * (sqrt((v1y-v2y)^2 + (v1x-v2x)^2));

f_damper_x_13_14 = damper_force *cos(theta_damper_after);
f_damper_y_13_14 = damper_force *sin(theta_damper_after);




theta_damper_before= atan2((v1y-v0y),(v1x-v0x));
% if v0x~=v1x
% theta_damper_before= atan((v0y-v1y)/(v0x-v1x));
% else
% theta_damper_before= 3.14/2;
% end




damper_force_before= -k_d * (sqrt((v0y-v1y)^2 + (v0x-v1x)^2));

f_damper_x_12_13 = damper_force_before *cos(theta_damper_before);
f_damper_y_12_13 = damper_force_before *sin(theta_damper_before);







a13_x = (  f_spring_x_13_14  +   f_damper_x_13_14  + f_spring_x_12_13 + f_damper_x_12_13 )/m;

a13_y = (  f_spring_y_13_14  +   f_damper_y_13_14 + f_spring_y_12_13 + f_damper_y_12_13 + m* (-9.81)  )/m;
